simulink library "Digital"  (R2017a)
settings: Solver=VariableStepAuto  StartTime=0.0  StopTime=10.0  RelTol=1e-3
settings Model: Creator=Di Russo  LastModifiedBy=Vraj M

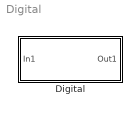
== system Digital ==
  Digital : Subsystem

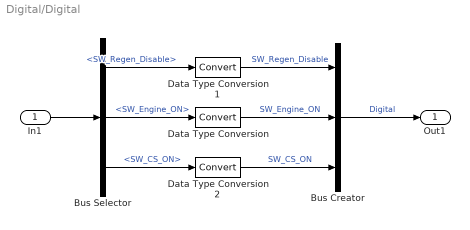
== system Digital/Digital ==
  In1 : Inport
  Bus Creator : BusCreator  Inputs=3
  Bus Selector : BusSelector  OutputSignals=Driver_Signals.SW_Regen_Disable,Driver_Signals.SW_Engine_ON,Driver_Signals.SW_CS_ON
  Data Type Conversion : DataTypeConversion
  Data Type Conversion1 : DataTypeConversion
  Data Type Conversion2 : DataTypeConversion
  Out1 : Outport
  wires:
  Bus Creator/1 -> Out1/1  "Digital"
  Data Type Conversion1/1 -> Bus Creator/1  "SW_Regen_Disable"
  Data Type Conversion2/1 -> Bus Creator/3  "SW_CS_ON"
  Data Type Conversion/1 -> Bus Creator/2  "SW_Engine_ON"
  Bus Selector/3 -> Data Type Conversion2/1  "<SW_CS_ON>"
  Bus Selector/2 -> Data Type Conversion/1  "<SW_Engine_ON>"
  Bus Selector/1 -> Data Type Conversion1/1  "<SW_Regen_Disable>"
  In1/1 -> Bus Selector/1
